simulink model "reduced_observer_for_secondpoles"  (R2021b)
settings: Solver=VariableStepAuto  StartTime=0.0  StopTime=2.5  RelTol=1e-3
undefined symbols (not defined in the file): A_1_1, A_2_2, Ao, B_1_1, Bo, Co, L_reduced2, Q1, Q2
settings Model: Creator=nima8  LastModifiedBy=nima8

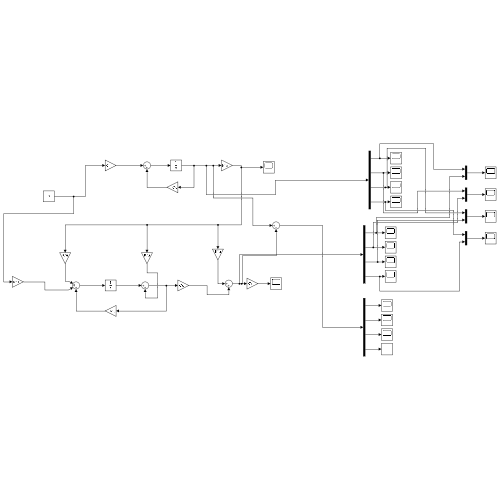
[thumbnail: Simulink's stored preview of the top-level diagram]
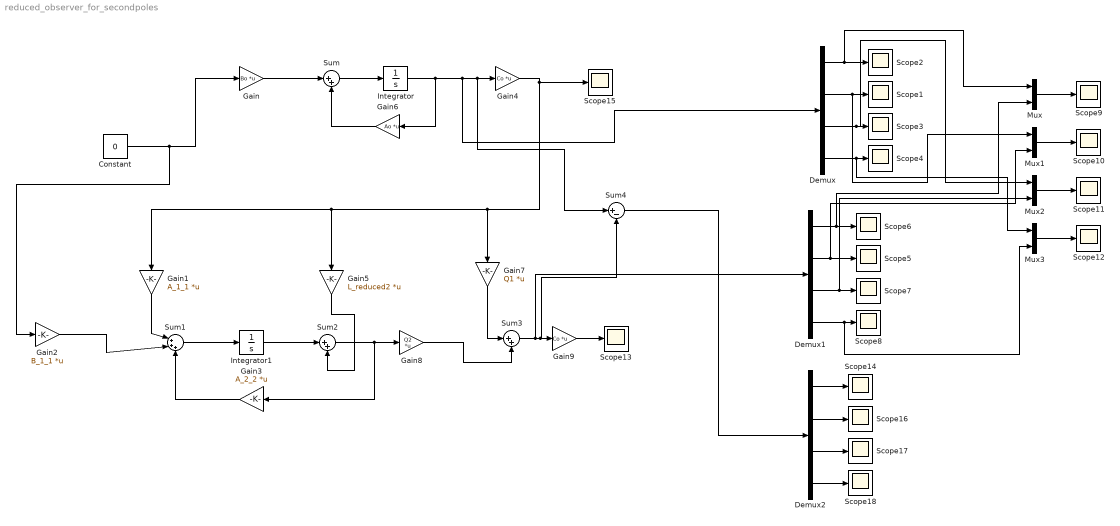
== system reduced_observer_for_secondpoles ==
  Constant : Constant  Value=0
  Demux : Demux
  Demux1 : Demux
  Demux2 : Demux
  Gain : Gain  Gain=Bo  Multiplication=Matrix(K*u)
  Gain1 : Gain  Gain=A_1_1  Multiplication=Matrix(K*u)
  Gain2 : Gain  Gain=B_1_1  Multiplication=Matrix(K*u)
  Gain3 : Gain  Gain=A_2_2  Multiplication=Matrix(K*u)
  Gain4 : Gain  Gain=Co  Multiplication=Matrix(K*u)
  Gain5 : Gain  Gain=L_reduced2  Multiplication=Matrix(K*u)
  Gain6 : Gain  Gain=Ao  Multiplication=Matrix(K*u)
  Gain7 : Gain  Gain=Q1  Multiplication=Matrix(K*u)
  Gain8 : Gain  Gain=Q2  Multiplication=Matrix(K*u)
  Gain9 : Gain  Gain=Co  Multiplication=Matrix(K*u)
  Integrator : Integrator  InitialCondition=[1 0.5 -1 2]
  Integrator1 : Integrator  InitialCondition=[-2 3 -2]
  Mux{,1..3} (4 alike) : Mux  Inputs=2
  Scope{1..18} (18 alike) : Scope
  Sum : Sum  Inputs=|++
  Sum1 : Sum  Inputs=|+++
  Sum2 : Sum  Inputs=|++
  Sum3 : Sum  Inputs=|++
  Sum4 : Sum  Inputs=|+-
  wires:
  Demux2/3 -> Scope17/1
  Gain8/1 -> Sum3/2
  Gain4/1 -> Scope15/1, Gain1/1, Gain5/1, Gain7/1
  Integrator1/1 -> Sum2/1
  Gain6/1 -> Sum/2
  Gain7/1 -> Sum3/1
  Sum4/1 -> Demux2/1
  Demux/3 -> Mux2/1, Scope3/1
  Demux2/1 -> Scope14/1
  Demux2/2 -> Scope16/1
  Sum/1 -> Integrator/1
  Mux1/1 -> Scope10/1
  Integrator/1 -> Demux/1, Sum4/1, Gain4/1, Gain6/1
  Sum2/1 -> Gain3/1, Gain8/1
  Sum3/1 -> Demux1/1, Sum4/2, Gain9/1
  Gain/1 -> Sum/1
  Gain1/1 -> Sum1/1
  Demux/4 -> Mux3/1, Scope4/1
  Mux3/1 -> Scope12/1
  Demux2/4 -> Scope18/1
  Gain9/1 -> Scope13/1
  Gain2/1 -> Sum1/2
  Demux1/4 -> Mux3/2, Scope8/1
  Gain3/1 -> Sum1/3
  Constant/1 -> Gain2/1, Gain/1
  Mux2/1 -> Scope11/1
  Demux/2 -> Mux1/1, Scope1/1
  Gain5/1 -> Sum2/2
  Demux1/3 -> Mux2/2, Scope7/1
  Demux1/2 -> Mux1/2, Scope5/1
  Demux/1 -> Mux/1, Scope2/1
  Demux1/1 -> Mux/2, Scope6/1
  Sum1/1 -> Integrator1/1
  Mux/1 -> Scope9/1
